simulink model "fz6_11"  (R2014a)
settings: Solver=ode45  StartTime=0.0  StopTime=2  RelTol=1e-3
libraries: commutil2 x4, commsink2 x2, commdigbbndam3 x2, commfilt2 x2, dspsigops x2, commchan3 x1, commrandsrc2 x1
settings Model: Creator=tzb  LastModifiedBy=tzb
settings DebuggingCC: SolverPrmCheckMsg=none  FrameProcessingCompatibilityMsg=none

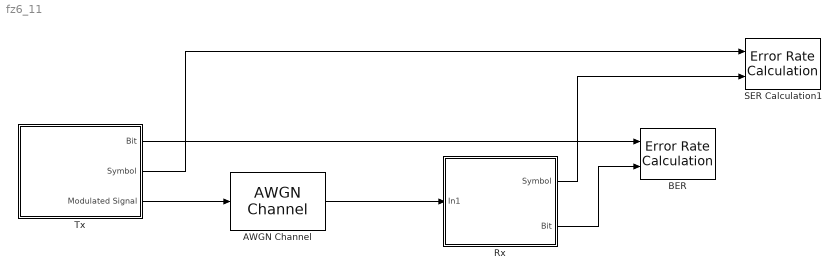
== system fz6_11 ==
  AWGN Channel : commchan3/AWGN Channel  InputProcessing=Inherited (this choice will be removed - see release notes)  seed=1234  noiseMode="Signal to noise ratio  (Es/No)"  EbNodB=10  EsNodB=SNR  SNRdB=10  bitsPerSym=1  Ps=0.5  Tsym=1/100000  variance=1
  BER : commsink2/Error Rate Calculation  N=0  st_delay=16  cp_mode=Entire frame  subframe=[]  PMode=Workspace  WsName=BER  RsMode2=off  stop=off  numErr=100  maxBits=1e6
  Rx : Subsystem
  SER Calculation1 : commsink2/Error Rate Calculation  N=0  st_delay=8  cp_mode=Entire frame  subframe=[]  PMode=Workspace  WsName=SER  RsMode2=off  stop=off  numErr=100  maxBits=1e6
  Tx : Subsystem
  wires:
  Tx/3(Modulated Signal) -> AWGN Channel/1
  AWGN Channel/1 -> Rx/1(In1)
  Rx/2(Bit) -> BER/2
  Rx/1(Symbol) -> SER Calculation1/2
  Tx/1(Bit) -> BER/1
  Tx/2(Symbol) -> SER Calculation1/1

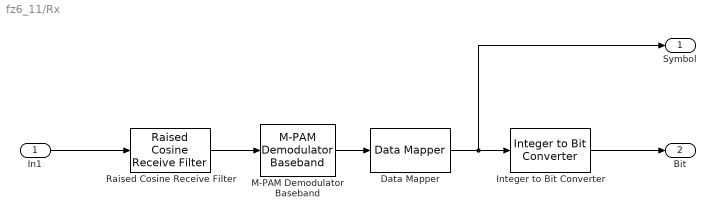
== system fz6_11/Rx ==
  In1 : Inport
  Data Mapper : commutil2/Data Mapper  MapMode=Gray to Binary  M=4  MapVec=[0 1 3 2 7 6 4 5]
  Integer to Bit Converter : commutil2/Integer to Bit Converter  nbits=2  signedInputValues=Unsigned  bitOrder=MSB first  outDtype=Inherit via internal rule
  M-PAM Demodulator Baseband : commdigbbndam3/M-PAM Demodulator Baseband  M=4  OutType=Integer  Dec=Gray  PowType=Min. distance between symbols  MinDist=2  AvgPow=1  PeakPow=1  outDtype1=Inherit via internal rule  outDtype2=Inherit via internal rule  denormFactorWordLen=16  prodOutWordLen=16  prodOutRoundingMode=Floor  prodOutOverflowMode=Wrap  sumWordLen=16
  Raised Cosine Receive Filter : commfilt2/Raised Cosine Receive Filter  filtType=Square root  N=10  filtSpan=2*(4)  currentFiltSpan=2*(4)  D=(2*(4))/2  R=0.25  sampMode=Mute  saveAsFlag=0  rateMode=Downsampling  downFactor=10  downOffset=0  framing=Enforce single-rate processing  InputProcessing=Columns as channels (frame based)  checkGain=Normalized  filterGain=1  checkCoeff=off  variableName=rcRxFilt  launchFVT=on  roundingMode=Floor  overflowMode=off
  Symbol : Outport
  Bit : Outport  Port=2
  wires:
  In1/1 -> Raised Cosine Receive Filter/1
  Data Mapper/1 -> Symbol/1, Integer to Bit Converter/1
  Raised Cosine Receive Filter/1 -> M-PAM Demodulator Baseband/1
  Integer to Bit Converter/1 -> Bit/1
  M-PAM Demodulator Baseband/1 -> Data Mapper/1

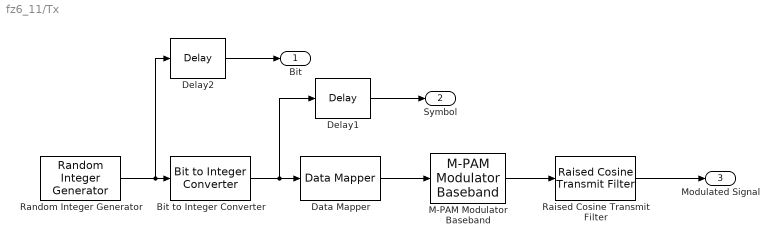
== system fz6_11/Tx ==
  Bit to Integer Converter : commutil2/Bit to Integer Converter  nbits=2  bitOrder=MSB first  signedOutputValues=Unsigned  outDtype=Inherit via internal rule  outDtypeSigned=Inherit via internal rule
  Data Mapper : commutil2/Data Mapper  MapMode=Binary to Gray  M=4  MapVec=[0 1 3 2 7 6 4 5]
  Delay1 : dspsigops/Delay  InputProcessing=Columns as channels (frame based)  dly_unit=Samples  delay=8  ic_detail=off  dif_ic_for_ch=off  dif_ic_for_dly=off  ic=0  reset_popup=None
  Delay2 : dspsigops/Delay  InputProcessing=Columns as channels (frame based)  dly_unit=Samples  delay=16  ic_detail=off  dif_ic_for_ch=off  dif_ic_for_dly=off  ic=0  reset_popup=None
  M-PAM Modulator Baseband : commdigbbndam3/M-PAM Modulator Baseband  M=4  InType=Integer  Enc=Gray  PowType=Min. distance between symbols  MinDist=2  AvgPow=1  PeakPow=1  outDtype=double  outWordLen=16  outUDDataType=sfix(16)  outFracLenMode=Best precision  outFracLen=15
  Raised Cosine Transmit Filter : commfilt2/Raised Cosine Transmit Filter  filtType=Square root  filtSpan=2*(4)  currentFiltSpan=2*(4)  D=(2*(4))/2  R=0.25  sampMode=Mute  saveAsFlag=0  N=10  framing=Enforce single-rate processing  InputProcessing=Columns as channels (frame based)  checkGain=Normalized  filterGain=1  checkCoeff=off  variableName=rcTxFilt  launchFVT=on  roundingMode=Floor  overflowMode=off
  Random Integer Generator : commrandsrc2/Random Integer Generator  mul=2  seed=37  Ts=1/200000  frameBased=on  sampPerFrame=200000  orient=off  outDataType=double
  Bit : Outport
  Symbol : Outport  Port=2
  Modulated Signal : Outport  Port=3
  wires:
  Bit to Integer Converter/1 -> Delay1/1, Data Mapper/1
  Random Integer Generator/1 -> Delay2/1, Bit to Integer Converter/1
  Delay2/1 -> Bit/1
  M-PAM Modulator Baseband/1 -> Raised Cosine Transmit Filter/1
  Raised Cosine Transmit Filter/1 -> Modulated Signal/1
  Data Mapper/1 -> M-PAM Modulator Baseband/1
  Delay1/1 -> Symbol/1
